simulink model "cross_vzmac_core"  (Simulink 7.9)
settings: Solver=ode45  StartTime=0.0  StopTime=2048*16+100  RelTol=1e-3
PreLoadFcn:
  | if ~exist('sync')
  |   sync=[1];
  | end
  | if ~exist('zin0')
  |   zin0=complex( ...
  |     floor(256*rand(1,15*2048+1))/128-1, ...
  |     floor(256*rand(1,15*2048+1))/128-1  ...
  |   );
  | end
  | if ~exist('zin1')
  |   zin1=complex( ...
  |     floor(256*rand(1,15*2048+1))/128-1, ...
  |     floor(256*rand(1,15*2048+1))/128-1  ...
  |   );
  | end
undefined symbols (not defined in the file or in its folder): A, B, PCIN, xlipgetpartsetting
libraries: xbsIndex_r4 x34
(part 1 of 6)
settings Model: Creator=mdexter  LastModifiedBy=mdexter

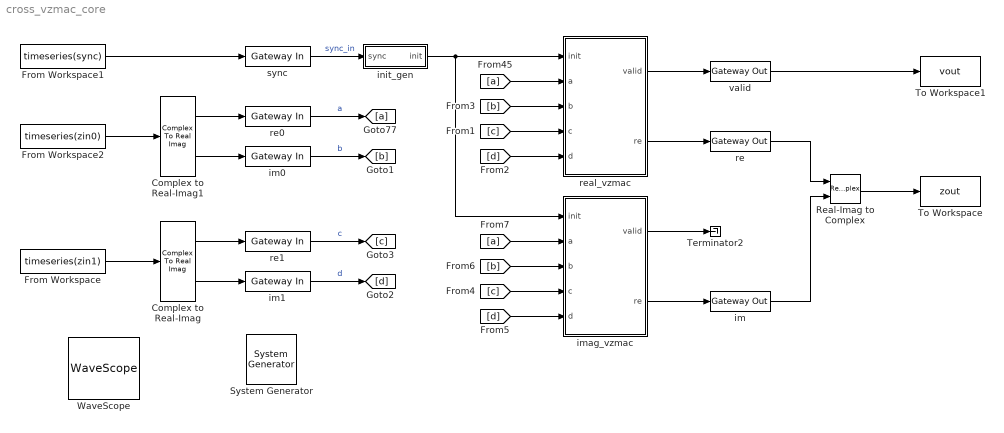
== system cross_vzmac_core ==
  " System Generator" : xbsIndex_r4/ System Generator  Tag=genX  xilinxfamily=virtex6  part=xc6vsx475t  speed=-1  package=ff1759  synthesis_tool=XST  clock_wrapper=Clock Enables  directory=./cross_vzmac_core  proj_type=Project Navigator  Synth_file=XST Defaults  Impl_file=ISE Defaults  testbench=off  simulink_period=1  sysclk_period=10  dcm_input_clock_period=10  incr_netlist=off  trim_vbits=Everywhere in SubSystem  dbl_ovrd=According to Block Masks  core_generation=According to Block Masks  run_coregen=off  deprecated_control=off  eval_field=0  block_type=sysgen
  Complex to Real-Imag : ComplexToRealImag
  Complex to Real-Imag1 : ComplexToRealImag
  From Workspace : FromWorkspace  VariableName=timeseries(zin1)  SampleTime=1  Interpolate=off  OutputAfterFinalValue=Setting to zero
  From Workspace1 : FromWorkspace  VariableName=timeseries(sync)  SampleTime=1  Interpolate=off  OutputAfterFinalValue=Setting to zero
  From Workspace2 : FromWorkspace  VariableName=timeseries(zin0)  SampleTime=1  Interpolate=off  OutputAfterFinalValue=Setting to zero
  Real-Imag to Complex : RealImagToComplex
  Terminator2 : Terminator
  To Workspace : ToWorkspace  VariableName=zout  SampleTime=-1
  To Workspace1 : ToWorkspace  VariableName=vout  SampleTime=-1
  WaveScope : xbsIndex_r4/WaveScope  block_type=wavescope
  im : xbsIndex_r4/Gateway Out  inherit_from_input=off  hdl_port=on  timing_constraint=None  locs_specified=off  LOCs={}  UseAsDAC=off  DACChannel='1'  block_type=gatewayout
      settings: xl_area=[0 0 0 0 21 0 0]
  im0 : xbsIndex_r4/Gateway In  gui_display_data_type=Fixed-point  arith_type="Signed  (2's comp)"  n_bits=8  bin_pt=7  preci_type=Single  exp_width=8  frac_width=24  quantization="Round  (unbiased: +/- Inf)"  overflow=Saturate  period=1  dbl_ovrd=off  timing_constraint=None  locs_specified=off  LOCs={}  UseAsADC=off  ADCChannel='1'  inherit_from_input=off  hdl_port=on  block_type=gatewayin
  im1 : xbsIndex_r4/Gateway In  gui_display_data_type=Fixed-point  arith_type="Signed  (2's comp)"  n_bits=8  bin_pt=7  preci_type=Single  exp_width=8  frac_width=24  quantization="Round  (unbiased: +/- Inf)"  overflow=Saturate  period=1  dbl_ovrd=off  timing_constraint=None  locs_specified=off  LOCs={}  UseAsADC=off  ADCChannel='1'  inherit_from_input=off  hdl_port=on  block_type=gatewayin
  imag_vzmac : Subsystem
  init_gen : Subsystem
  re : xbsIndex_r4/Gateway Out  inherit_from_input=off  hdl_port=on  timing_constraint=None  locs_specified=off  LOCs={}  UseAsDAC=off  DACChannel='1'  block_type=gatewayout
      settings: xl_area=[0 0 0 0 21 0 0]
  re0 : xbsIndex_r4/Gateway In  gui_display_data_type=Fixed-point  arith_type="Signed  (2's comp)"  n_bits=8  bin_pt=7  preci_type=Single  exp_width=8  frac_width=24  quantization="Round  (unbiased: +/- Inf)"  overflow=Saturate  period=1  dbl_ovrd=off  timing_constraint=None  locs_specified=off  LOCs={}  UseAsADC=off  ADCChannel='1'  inherit_from_input=off  hdl_port=on  block_type=gatewayin
  re1 : xbsIndex_r4/Gateway In  gui_display_data_type=Fixed-point  arith_type="Signed  (2's comp)"  n_bits=8  bin_pt=7  preci_type=Single  exp_width=8  frac_width=24  quantization="Round  (unbiased: +/- Inf)"  overflow=Saturate  period=1  dbl_ovrd=off  timing_constraint=None  locs_specified=off  LOCs={}  UseAsADC=off  ADCChannel='1'  inherit_from_input=off  hdl_port=on  block_type=gatewayin
  real_vzmac : Subsystem
  sync : xbsIndex_r4/Gateway In  gui_display_data_type=Boolean  arith_type=Boolean  n_bits=8  bin_pt=7  preci_type=Single  exp_width=8  frac_width=24  quantization="Round  (unbiased: +/- Inf)"  overflow=Saturate  period=1  dbl_ovrd=off  timing_constraint=None  locs_specified=off  LOCs={}  UseAsADC=off  ADCChannel='1'  inherit_from_input=off  hdl_port=on  block_type=gatewayin
  valid : xbsIndex_r4/Gateway Out  inherit_from_input=off  hdl_port=on  timing_constraint=None  locs_specified=off  LOCs={}  UseAsDAC=off  DACChannel='1'  block_type=gatewayout
      settings: xl_area=[0 0 0 0 21 0 0]
  wires:
  re/1 -> Real-Imag to Complex/1
  re0/1 -> [a]  "a"
  real_vzmac/1(valid) -> valid/1
  valid/1 -> To Workspace1/1
  real_vzmac/2(re) -> re/1
  im0/1 -> [b]  "b"
  re1/1 -> [c]  "c"
  im1/1 -> [d]  "d"
  [a] -> real_vzmac/2(a)
  [c] -> real_vzmac/4(c)
  [b] -> real_vzmac/3(b)
  [d] -> real_vzmac/5(d)
  Complex to Real-Imag/2 -> im1/1
  Complex to Real-Imag/1 -> re1/1
  From Workspace1/1 -> sync/1
  sync/1 -> init_gen/1(sync)  "sync_in"
  init_gen/1(init) -> real_vzmac/1(init), imag_vzmac/1(init)
  From Workspace/1 -> Complex to Real-Imag/1
  im/1 -> Real-Imag to Complex/2
  imag_vzmac/1(valid) -> Terminator2/1
  imag_vzmac/2(re) -> im/1
  [a] -> imag_vzmac/2(a)
  [c] -> imag_vzmac/4(c)
  [b] -> imag_vzmac/3(b)
  [d] -> imag_vzmac/5(d)
  Real-Imag to Complex/1 -> To Workspace/1
  From Workspace2/1 -> Complex to Real-Imag1/1
  Complex to Real-Imag1/1 -> re0/1
  Complex to Real-Imag1/2 -> im0/1
